simulink model "Subsystem"  (R2020b)
settings: Solver=FixedStepAuto  StartTime=0.0  StopTime=10.0  FixedStep=1  MaxStep=0.01  RelTol=1e-3
settings Model: Creator=lalit  LastModifiedBy=lalit
settings DataIOCC: SaveOutput=off  SaveTime=off

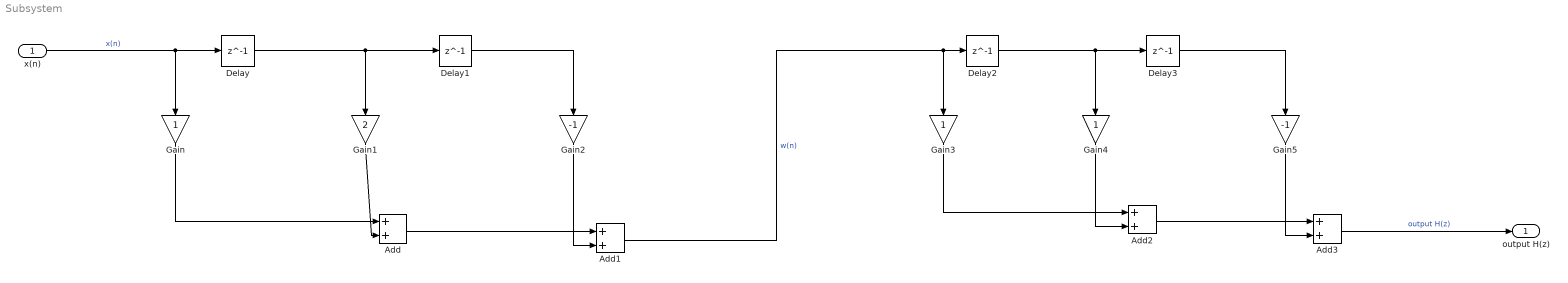
== system Subsystem ==
  x(n) : Inport  OutDataTypeStr=double  PortDimensions=[1 1]  SampleTime=[1,0]
  Add{,1..3} (4 alike) : Sum
  Delay{,1..3} (4 alike) : Delay  DelayLength=1
  Gain : Gain
  Gain1 : Gain  Gain=2
  Gain2 : Gain  Gain=-1
  Gain3 : Gain
  Gain4 : Gain
  Gain5 : Gain  Gain=-1
  output H(z) : Outport  OutDataTypeStr=double  PortDimensions=[1 1]  SampleTime=[1,0]
  wires:
  Delay2/1 -> Delay3/1, Gain4/1
  Gain4/1 -> Add2/2
  Add3/1 -> output H(z)/1  "output H(z)"
  Add2/1 -> Add3/1
  Delay1/1 -> Gain2/1
  Delay/1 -> Delay1/1, Gain1/1
  Add1/1 -> Delay2/1, Gain3/1  "w(n)"
  Gain1/1 -> Add/2
  Delay3/1 -> Gain5/1
  Add/1 -> Add1/1
  Gain/1 -> Add/1
  x(n)/1 -> Delay/1, Gain/1  "x(n)"
  Gain2/1 -> Add1/2
  Gain3/1 -> Add2/1
  Gain5/1 -> Add3/2
